simulink model "torbsc_m"  (Simulink 8.5)
settings: Solver=ode45  SolverMode=SingleTasking  StartTime=0.0  StopTime=999999  MaxStep=10  RelTol=1e-3  AbsTol=1e-3
values from neighbouring files (symbols this model uses):
  U = st_Varia('ShortNames')    [torbk2_i.m]    (also in torbsc_i.m)
  x0 = [0.00001;zeros(NumCel-1,1);zeros(NumCel,1);0.0000005*ones(NumCel,1);zeros(NumCel,1);zeros(NumCel,1);0;0;0;0;0;zeros(NumCel,1);0.0002*ones(NumCel,1);zeros(NumCel,1);zeros(NumCel,1);zeros(NumCel,1);zeros(NumCel,1)]    [torbk2_i.m]    (also in torbk2_s.m = x0; torbsc_i.m; torbsc_s.m = x0)
undefined symbols (not defined in the file or in its folder): B
settings Model: Creator=M.Sparnaaij  LastModifiedBy=Martijn
settings DataIOCC: LimitDataPoints=off  SaveOutput=off  SaveTime=off  SignalLoggingName=sigsOut
settings OptimizationCC: BooleanDataType=off
settings DebuggingCC: SaveWithParameterizedLinksMsg=none  SignalResolutionControl=TryResolveAllWithWarning  MultiTaskDSMMsg=warning  MultiTaskCondExecSysMsg=none  FcnCallInpInsideContextMsg=EnableAllAsWarning  StrictBusMsg=None
settings HardwareCC: TargetUnknown=on

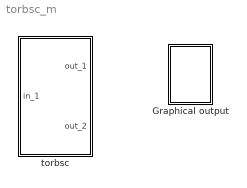
== system torbsc_m ==
  Graphical output : Subsystem
      settings: OpenFcn=torbsc_g
      mask Display:
      | plot(0,0,100,100,[80,20,20],[20,20,80],[80,69,60,52,45,39,33,28,24,20],[65,65,64,61,57,52,45,37,30,20])
      | disp('');
      | text(100,100,'torbsc', 'horizontalAlignment', 'right', 'verticalAlignment', 'top');
  torbsc : Subsystem  Description=This model calculates the aeration and degassifying with a packed column aerator. The influent carbon dioxide concentration is calculated on the basis of the bicarbonate concentration, the pH, the EGV and the water temperature, so these parameters must always be filled out in the 'Water quality parameters' block.
      mask init:
      | filenaam='.\StimelaData\Packed_column_aerator_sc.mat';
      | 
      | [Pn,Fn,Fext]=Fileprop(filenaam);
      | 
      | errstr = st_UniqName(filenaam,'filenaam=''','SubSystem','OpenFcn');
      | if errstr, error([errstr 'The filename "' filenaam '" is already in use. Choose a different filename.']), end
      | 
      | P = torbsc_p(filenaam);
      | [B,x0,U]=torbsc_i(filenaam);
      settings: OpenFcn=|
      | filenaam='.\StimelaData\Packed_column_aerator_sc.mat';
      | st_ParameterInput('init',gcb,filenaam,'torbsc');
      mask Display:
      | plot(0,0,100,100,[20,20],[20,80],[80,80],[20,80],[20,80,20,80,20],[30,70,70,30,30],[80,20],[28,28],[50,44,34,27,23,20],[90,90,89,87,84,80],[50,44,34,27,23,20],[10,10,11,13,16,20],[50,56,66,73,77,80],[90,90,89,87,84,80],[50,56,66,73,77,80],[10,10,11,13,16,20],[21,20],[82,80],[10,50,50,10],[82,82,80,80],[58,50,42],[76,80,76],[50,35,45,45],[99,94,94,90],[50,65,55,55],[99,94,94,90],[45,45],[3,10],[55,55],[3,10])
      | disp('')
      | text(50,50,'torbsc', 'horizontalAlignment', 'center', 'verticalAlignment', 'middle');
      | text(50,0,Fn, 'horizontalAlignment', 'center', 'verticalAlignment', 'base');

== system torbsc_m/Graphical output ==
  note: plotten

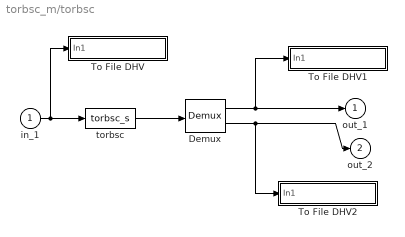
== system torbsc_m/torbsc ==
  in_1 : Inport
  Demux : Demux  Outputs=[U.Number B.Measurements]
  To File DHV : Subsystem  mask(To File DHV){naam=[filenaam(1:length(filenaam)-4) '_in.sti']}
      mask prompts: naam "Naam van bestand"
      mask init:
      | set_param([gcb '/To File'],'Filename',naam);
      mask Display: disp(naam)
  To File DHV1 : Subsystem  mask(To File DHV){naam=[filenaam(1:length(filenaam)-4) '_out.sti']}
      mask prompts: naam "Naam van bestand"
      mask init:
      | set_param([gcb '/To File'],'Filename',naam);
      mask Display: disp(naam)
  To File DHV2 : Subsystem  mask(To File DHV){naam=[filenaam(1:length(filenaam)-4) '_EM.sti']}
      mask prompts: naam "Naam van bestand"
      mask init:
      | set_param([gcb '/To File'],'Filename',naam);
      mask Display: disp(naam)
  torbsc : S-Function  FunctionName=torbsc_s  Parameters=B,x0,U,P
  out_1 : Outport  InitialOutput=0
  out_2 : Outport  Port=2  InitialOutput=0
  wires:
  in_1/1 -> To File DHV/1(In1), torbsc/1
  Demux/2 -> To File DHV2/1(In1), out_2/1
  Demux/1 -> To File DHV1/1(In1), out_1/1
  torbsc/1 -> Demux/1

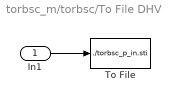
== system torbsc_m/torbsc/To File DHV ==
  In1 : Inport
  To File : ToFile  Filename=./torbsc_p_in.sti  MatrixName=torbscin
  wires:
  In1/1 -> To File/1

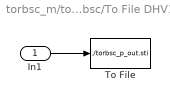
== system torbsc_m/torbsc/To File DHV1 ==
  In1 : Inport
  To File : ToFile  Filename=./torbsc_p_out.sti  MatrixName=torbscout
  wires:
  In1/1 -> To File/1

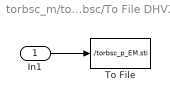
== system torbsc_m/torbsc/To File DHV2 ==
  In1 : Inport
  To File : ToFile  Filename=./torbsc_p_EM.sti  MatrixName=torbscEM
  wires:
  In1/1 -> To File/1
